simulink model "Ex4_6"  (R2016b)
settings: Solver=VariableStepAuto  StartTime=0.0  StopTime=100  RelTol=1e-3
values from neighbouring files (symbols this model uses):
  alpha = 0.005    [ex4_3_init.m]    (also in ex4_5_init.m = 12.87)
  Gaf = 1.273    [ex4_3_init.m]    (also in ex4_5_init.m = 0.8858)
  Gr = 4.3    [ex4_5_init.m]
  I_set = 0    [ex4_5_init.m]
  Ia_0 = 0    [ex4_5_init.m]
  Ia_ol = 3*Ia_rat    (= 612)    [ex4_5_init.m]
  If_0 = 4    [ex4_5_init.m]
  Kp_i = 0.22    [ex4_3_init.m]    (also in ex4_5_init.m = 1000)
  Kp_w = 10000000    [ex4_3_init.m]    (also in ex4_5_init.m = 1000)
  La = 0.002    [ex4_3_init.m]    (also in ex4_5_init.m = 0.235783633842)
  m = 142.7    [ex4_3_init.m]    (also in ex4_5_init.m = 110000)
  Ra = 0.05    [ex4_3_init.m]    (also in ex4_5_init.m = 0.1442)
  Rf = 200    [ex4_3_init.m]    (also in ex4_5_init.m = 375)
  Rs_0 = 2.3068    [ex4_5_init.m]
  Rs_on = 0    [ex4_5_init.m]
  Rs_wm = 2.3068/415    (= 0.00555855421687)    [ex4_5_init.m]
  Rw = 0.46    [ex4_5_init.m]
  tdc = 0.01    [ex4_5_init.m]
  Ti_i = 5.4    [ex4_3_init.m]    (also in ex4_5_init.m = 50)
  Ti_i_lim = 1500    [ex4_5_init.m]
  Ti_w = 0.01    [ex4_3_init.m]    (also in ex4_5_init.m = 15)
  Ti_w_lim = 50    [ex4_5_init.m]
  Ua = 1500    [ex4_5_init.m]
  Uf = 220    [ex4_3_init.m]    (also in ex4_5_init.m = 1500)
  V_set = 44    [ex4_5_init.m]
undefined symbols (not defined in the file or in its folder): sigbuilder_block
libraries: simulink x8
settings Model: Creator=Niels  LastModifiedBy=Niels

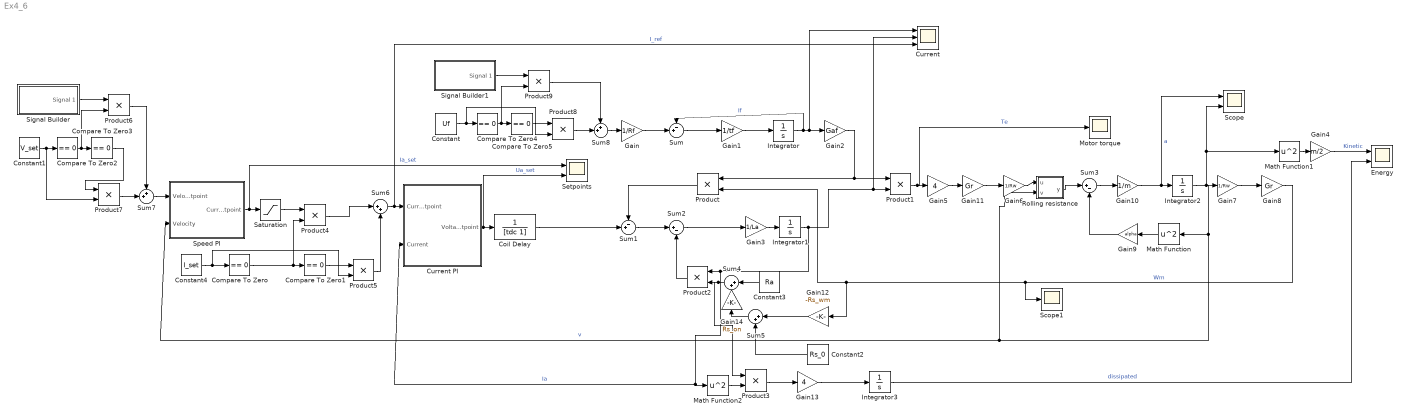
== system Ex4_6 ==
  Coil Delay : TransferFcn  Denominator=[tdc 1]
  Compare To Zero{,1..5} (6 alike) : simulink/Logic and Bit Operations/Compare To Zero  relop===  OutDataTypeStr=boolean
  Constant : Constant  Value=Uf
  Constant1 : Constant  Value=V_set
  Constant2 : Constant  Value=Rs_0
  Constant3 : Constant  Value=Ra
  Constant4 : Constant  Value=I_set
  Current : Scope  NumInputPorts=3
  Current PI : Subsystem
  Energy : Scope  NumInputPorts=2
  Gain : Gain  Gain=1/Rf
  Gain1 : Gain  Gain=1/tf
  Gain10 : Gain  Gain=1/m
  Gain11 : Gain  Gain=Gr
  Gain12 : Gain  Gain=-Rs_wm
  Gain13 : Gain  Gain=4
  Gain14 : Gain  Gain=Rs_on
  Gain2 : Gain  Gain=Gaf
  Gain3 : Gain  Gain=1/La
  Gain4 : Gain  Gain=m/2
  Gain5 : Gain  Gain=4
  Gain6 : Gain  Gain=1/Rw
  Gain7 : Gain  Gain=1/Rw
  Gain8 : Gain  Gain=Gr
  Gain9 : Gain  Gain=alpha
  Integrator : Integrator  InitialCondition=If_0
  Integrator1 : Integrator  InitialCondition=Ia_0
  Integrator2 : Integrator
  Integrator3 : Integrator
  Math Function : Math  Operator=square  SaturateOnIntegerOverflow=on
  Math Function1 : Math  Operator=square  SaturateOnIntegerOverflow=on
  Math Function2 : Math  Operator=square  SaturateOnIntegerOverflow=on
  Motor torque : Scope
  Product{,1..9} (10 alike) : Product
  Rolling resistance : MATLAB Function  TreatAsAtomicUnit=on
  Saturation : Saturate  UpperLimit=Ia_ol  LowerLimit=-Ia_ol
  Scope : Scope  NumInputPorts=2
  Scope1 : Scope
  Setpoints : Scope  NumInputPorts=2
  Signal Builder : Subsystem  Tag=STV Subsys  LoadFcn=sigbuilder_block('load');  StartFcn=sigbuilder_block('start');  StopFcn=sigbuilder_block('stop');  ClipboardFcn=sigbuilder_block('clipboard');  mask(Sigbuilder block){tuvar=[0:10]}
      mask help: Simulink:masks:SigbuilderBlock_MD
      mask init:
      | if ~strcmp(get_param(bdroot(gcbh),'SimulationStatus'),'stopped') tuvar = sigbuilder_block('maskInit'); end
      settings: CopyFcn=sigbuilder_block('copy');  DeleteFcn=sigbuilder_block('delete');  ModelCloseFcn=sigbuilder_block('modelClose');  PreSaveFcn=sigbuilder_block('preSave');  PauseFcn=sigbuilder_block('pause');  ContinueFcn=sigbuilder_block('continue');  NameChangeFcn=sigbuilder_block('namechange');  OpenFcn=sigbuilder_block('open',[437.6 199.2 550.4 400 ]);  CloseFcn=sigbuilder_block('close');
      mask Display: plot(0, 0, 100, 100,[2, 2, 32, 32, 2], [68, 8, 8, 68, 68],[32, 2], [38, 38], [32, 19, 2],[53, 60, 44], [32, 17, 17, 2],[16, 16, 31, 31]);txt = getActiveGroup(gcbh);text(2, 100, txt,'verticalAlignment', 'top');
  Signal Builder1 : Subsystem  Tag=STV Subsys  LoadFcn=sigbuilder_block('load');  StartFcn=sigbuilder_block('start');  StopFcn=sigbuilder_block('stop');  ClipboardFcn=sigbuilder_block('clipboard');  mask(Sigbuilder block){tuvar=[0:10]}
      mask help: Simulink:masks:SigbuilderBlock_MD
      mask init:
      | if ~strcmp(get_param(bdroot(gcbh),'SimulationStatus'),'stopped') tuvar = sigbuilder_block('maskInit'); end
      settings: CopyFcn=sigbuilder_block('copy');  DeleteFcn=sigbuilder_block('delete');  ModelCloseFcn=sigbuilder_block('modelClose');  PreSaveFcn=sigbuilder_block('preSave');  PauseFcn=sigbuilder_block('pause');  ContinueFcn=sigbuilder_block('continue');  NameChangeFcn=sigbuilder_block('namechange');  OpenFcn=sigbuilder_block('open',[437.6 199.2 550.4 400 ]);  CloseFcn=sigbuilder_block('close');
      mask Display: plot(0, 0, 100, 100,[2, 2, 32, 32, 2], [68, 8, 8, 68, 68],[32, 2], [38, 38], [32, 19, 2],[53, 60, 44], [32, 17, 17, 2],[16, 16, 31, 31]);txt = getActiveGroup(gcbh);text(2, 100, txt,'verticalAlignment', 'top');
  Speed PI : Subsystem
  Sum : Sum  Inputs=-+|
  Sum1 : Sum  Inputs=-+|
  Sum2 : Sum  Inputs=|+-
  Sum3 : Sum  Inputs=|+-
  Sum4 : Sum  Inputs=|++
  Sum5 : Sum  Inputs=|++
  Sum6 : Sum  Inputs=|++
  Sum7 : Sum  Inputs=++|
  Sum8 : Sum  Inputs=++|
  wires:
  Gain/1 -> Sum/2
  Sum/1 -> Gain1/1
  Gain1/1 -> Integrator/1
  Integrator/1 -> Current/1, Gain2/1, Sum/1  "If"
  Gain3/1 -> Integrator1/1
  Integrator1/1 -> Math Function2/1, Current PI/2(Current), Product2/1, Current/2, Product1/2  "Ia"
  Coil Delay/1 -> Sum1/2
  Product/1 -> Sum1/1
  Gain2/1 -> Product/1, Product1/1
  Product1/1 -> Motor torque/1, Gain5/1  "Te"
  Gain5/1 -> Gain11/1
  Integrator2/1 -> Rolling resistance/2(v), Speed PI/2(Velocity), Math Function/1, Gain7/1, Math Function1/1, Scope/2  "v"
  Gain7/1 -> Gain8/1
  Gain8/1 -> Scope1/1, Gain12/1, Product/2  "Wm"
  Math Function/1 -> Gain9/1
  Gain9/1 -> Sum3/2
  Rolling resistance/1(y) -> Sum3/1
  Gain10/1 -> Scope/1, Integrator2/1  "a"
  Sum3/1 -> Gain10/1
  Sum2/1 -> Gain3/1
  Sum1/1 -> Sum2/1
  Gain11/1 -> Gain6/1
  Gain6/1 -> Rolling resistance/1(u)
  Constant3/1 -> Sum4/1
  Sum5/1 -> Gain14/1
  Gain12/1 -> Sum5/1
  Constant2/1 -> Sum5/2
  Sum4/1 -> Product3/1, Product2/2
  Product2/1 -> Sum2/2
  Math Function1/1 -> Gain4/1
  Gain4/1 -> Energy/1  "Kinetic"
  Math Function2/1 -> Product3/2
  Product3/1 -> Gain13/1
  Gain13/1 -> Integrator3/1
  Integrator3/1 -> Energy/2  "dissipated"
  Current PI/1(Voltage Setpoint) -> Setpoints/2, Coil Delay/1  "Ua_set"
  Speed PI/1(Current Setpoint) -> Setpoints/1, Saturation/1  "Ia_set"
  Constant4/1 -> Product5/2, Compare To Zero/1
  Saturation/1 -> Product4/1
  Compare To Zero/1 -> Compare To Zero1/1, Product4/2
  Compare To Zero1/1 -> Product5/1
  Sum6/1 -> Current/3, Current PI/1(Current Setpoint)  "I_ref"
  Product4/1 -> Sum6/1
  Product5/1 -> Sum6/2
  Compare To Zero2/1 -> Product6/2, Compare To Zero3/1
  Constant1/1 -> Product7/2, Compare To Zero2/1
  Sum7/1 -> Speed PI/1(Velocity Setpoint)
  Signal Builder/1(Signal 1) -> Product6/1
  Product6/1 -> Sum7/1
  Product7/1 -> Sum7/2
  Compare To Zero3/1 -> Product7/1
  Compare To Zero4/1 -> Product9/2, Compare To Zero5/1
  Constant/1 -> Product8/2, Compare To Zero4/1
  Compare To Zero5/1 -> Product8/1
  Signal Builder1/1(Signal 1) -> Product9/1
  Product8/1 -> Sum8/2
  Product9/1 -> Sum8/1
  Sum8/1 -> Gain/1
  Gain14/1 -> Sum4/2

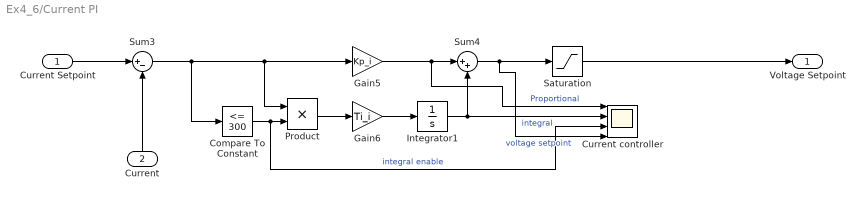
== system Ex4_6/Current PI ==
  Current Setpoint : Inport
  Current : Inport  Port=2
  Compare To Constant : simulink/Logic and Bit Operations/Compare To Constant  relop=<=  const=300  OutDataTypeStr=boolean
  Current controller : Scope  NumInputPorts=4
  Gain5 : Gain  Gain=Kp_i
  Gain6 : Gain  Gain=Ti_i
  Integrator1 : Integrator  LimitOutput=on  UpperSaturationLimit=Ti_i_lim  LowerSaturationLimit=-Ti_i_lim
  Product : Product
  Saturation : Saturate  UpperLimit=Ua  LowerLimit=-Ua
  Sum3 : Sum  Inputs=|+-
  Sum4 : Sum  Inputs=|++
  Voltage Setpoint : Outport
  wires:
  Sum3/1 -> Compare To Constant/1, Product/1, Gain5/1
  Current Setpoint/1 -> Sum3/1
  Sum4/1 -> Current controller/4, Saturation/1  "voltage setpoint"
  Current/1 -> Sum3/2
  Integrator1/1 -> Current controller/2, Sum4/2  "integral"
  Gain6/1 -> Integrator1/1
  Gain5/1 -> Current controller/1, Sum4/1  "Proportional"
  Saturation/1 -> Voltage Setpoint/1
  Product/1 -> Gain6/1
  Compare To Constant/1 -> Current controller/3, Product/2  "integral enable"

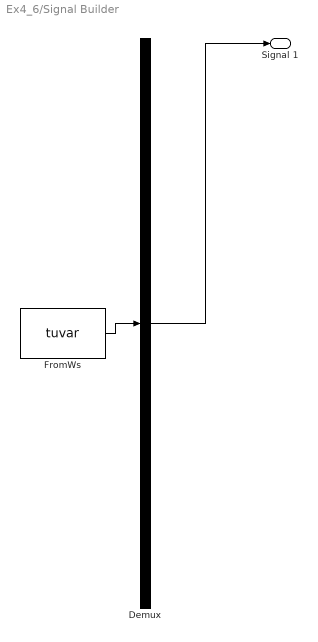
== system Ex4_6/Signal Builder ==
  Demux : Demux  Tag=STV Demux  Outputs=1
  FromWs : FromWorkspace  Tag=STV FromWs  VariableName=tuvar  SampleTime=0
      SigBuilderData=|
      | common.afterFinalStr = 'Extrapolate'
      | common.sampleTime = 0
      | dataSet.timeRange = [0 200]
      | dataSet.name = 'Group 1'
      | sbobj.Groups.Name = 'Group 1'
      | sbobj.Groups.Signals.Name = 'Signal 1'
      | sbobj.Groups.Signals.XData = [0 110 110 200]
      | sbobj.Groups.Signals.YData = [44 44 50 50]
      | sbobj.Groups.TimeRange = [0 200]
  Signal 1 : Outport  Tag=STV Outport
  wires:
  Demux/1 -> Signal 1/1
  FromWs/1 -> Demux/1

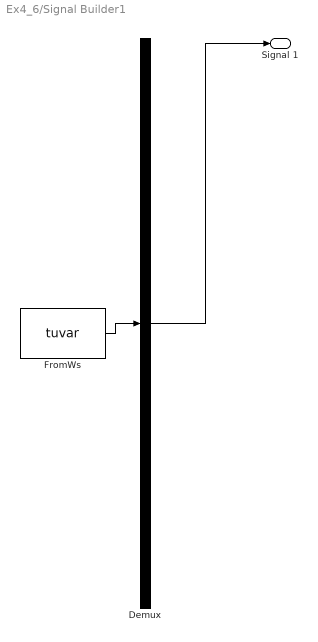
== system Ex4_6/Signal Builder1 ==
  Demux : Demux  Tag=STV Demux  Outputs=1
  FromWs : FromWorkspace  Tag=STV FromWs  VariableName=tuvar  SampleTime=0
      SigBuilderData=|
      | common.afterFinalStr = 'Extrapolate'
      | common.sampleTime = 0
      | dataSet.timeRange = [0 200]
      | dataSet.name = 'Group 1'
      | sbobj.Groups.Name = 'Group 1'
      | sbobj.Groups.Signals.Name = 'Signal 1'
      | sbobj.Groups.Signals.XData = [0 90 90 200]
      | sbobj.Groups.Signals.YData = [1500 1500 1200 1200]
      | sbobj.Groups.TimeRange = [0 200]
  Signal 1 : Outport  Tag=STV Outport
  wires:
  Demux/1 -> Signal 1/1
  FromWs/1 -> Demux/1

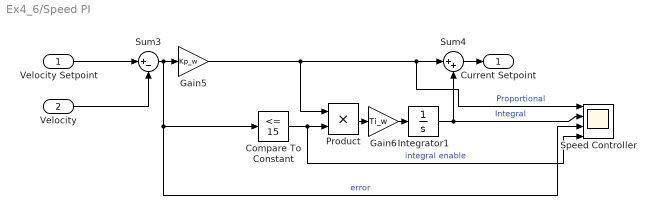
== system Ex4_6/Speed PI ==
  Velocity Setpoint : Inport
  Velocity : Inport  Port=2
  Compare To Constant : simulink/Logic and Bit Operations/Compare To Constant  relop=<=  const=15  OutDataTypeStr=boolean
  Gain5 : Gain  Gain=Kp_w
  Gain6 : Gain  Gain=Ti_w
  Integrator1 : Integrator  LimitOutput=on  UpperSaturationLimit=Ti_w_lim  LowerSaturationLimit=-Ti_w_lim
  Product : Product
  Speed Controller : Scope  NumInputPorts=4
  Sum3 : Sum  Inputs=|+-
  Sum4 : Sum  Inputs=|++
  Current Setpoint : Outport
  wires:
  Gain6/1 -> Integrator1/1
  Sum4/1 -> Current Setpoint/1
  Velocity/1 -> Sum3/2
  Sum3/1 -> Compare To Constant/1, Speed Controller/3, Gain5/1  "error"
  Velocity Setpoint/1 -> Sum3/1
  Gain5/1 -> Speed Controller/1, Sum4/1, Product/1  "Proportional"
  Integrator1/1 -> Speed Controller/2, Sum4/2  "Integral"
  Product/1 -> Gain6/1
  Compare To Constant/1 -> Speed Controller/4, Product/2  "integral enable"

== matlab function Ex4_6/Rolling resistance ==
  data: u input; y output; Frol parameter; v input
function y = fcn(u,Frol,v)
y = u - Frol;
if u <= Frol && abs(v) <= 0.01
    y = 0;
end
